simulink model "navigationstates"  (R2013b)
settings: Solver=FixedStepDiscrete  SolverMode=SingleTasking  StartTime=0.0  StopTime=inf  FixedStep=0.002  RelTol=1e-3
libraries: arduinolib x8, simulink x3
settings Model: SimulationMode=external  ExtModeTrigDuration=2  Creator=gcampa  LastModifiedBy=Joshua
settings DataIOCC: SignalLoggingSaveFormat=ModelDataLogs  SaveOutput=off  SaveTime=off
settings OptimizationCC: ExpressionDepthLimit=2147483647  OptimizeModelRefInitCode=on  LifeSpan=1
settings DebuggingCC: SolverPrmCheckMsg=none  MultiTaskDSMMsg=warning  MultiTaskCondExecSysMsg=none  FcnCallInpInsideContextMsg=EnableAllAsWarning  StateNameClashWarn=warning  StrictBusMsg=None
settings HardwareCC: ProdBitPerInt=16  ProdBitPerPointer=16  ProdIntDivRoundTo=Zero  ProdEndianess=LittleEndian  ProdWordSize=8  ProdHWDeviceType=Atmel->AVR
settings RTWCC: SystemTargetFile=realtime.tlc  GenerateMakefile=off  TemplateMakefile=realtime.tmf  Description=Real-Time Toolbox  RTWVerbose=off  ProcessScript=realtime_make_rtw_hook  IncludeERTFirstTime=on
settings CodeAppCC: CustomSymbolStrType=$N$R$M  InternalIdentifier=Classic
settings STFCustomTargetCC: TargetLibSuffix=.a  CodeReplacementLibrary=None  GenerateSampleERTMain=on  ERTCustomFileBanners=on  SupportNonInlinedSFcns=off  SupportVariableSizeSignals=on  MATLABClassNameForMDSCustomization=Simulink.SoftwareTarget.ERTCustomization  GRTInterface=off  SystemTargetFile=realtime.tlc
settings ERTTargetCC: GenerateSampleERTMain=on  ParMdlRefBuildCompliant=off  CompOptLevelCompliant=off  ConcurrentExecutionCompliant=off  CombineOutputUpdateFcns=off  ERTFirstTimeCompliant=off  SupportContinuousTime=on  SupportVariableSizeSignals=on  ModelStepFunctionPrototypeControlCompliant=off  CPPClassGenCompliant=off  ExtModeTransport=3  ExtModeMexFile=ext_serial_win32_comm  ExtModeMexArgs=0 1 9600  InlinedParameterPlacement=NonHierarchical  ERTSrcFileBannerTemplate=realtime_code_template.cgt  ERTHdrFileBannerTemplate=realtime_code_template.cgt  ERTDataSrcFileTemplate=realtime_code_template.cgt  ERTDataHdrFileTemplate=realtime_code_template.cgt  ERTCustomFileTemplate=realtime_file_process.tlc

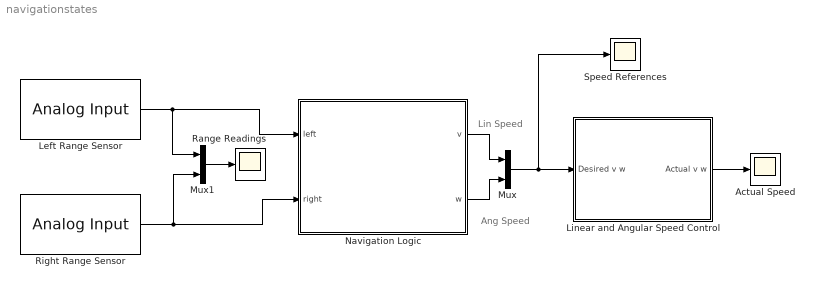
== system navigationstates ==
  note: Ang Speed
  note: Lin Speed
  Actual Speed : Scope
      settings: YMin=34.7  YMax=36
  Left Range Sensor : arduinolib/Analog Input  pinNumber=1  sampleTime=0.05
  Linear and Angular Speed Control : Subsystem
  Mux : Mux  Inputs=2
  Mux1 : Mux  Inputs=2
  Navigation Logic : Stateflow chart  TreatAsAtomicUnit=on
  Range Readings : Scope
      settings: YMin=34.7  YMax=36  SaveName=ScopeData3
  Right Range Sensor : arduinolib/Analog Input  pinNumber=0  sampleTime=0.05
  Speed References : Scope
      settings: YMin=34.7  YMax=36  SaveName=ScopeData2
  wires:
  Navigation Logic/1(v) -> Mux/1
  Mux/1 -> Speed References/1, Linear and Angular Speed Control/1(Desired v w)
  Linear and Angular Speed Control/1(Actual v w) -> Actual Speed/1
  Navigation Logic/2(w) -> Mux/2
  Right Range Sensor/1 -> Navigation Logic/2(right), Mux1/2
  Left Range Sensor/1 -> Navigation Logic/1(left), Mux1/1
  Mux1/1 -> Range Readings/1

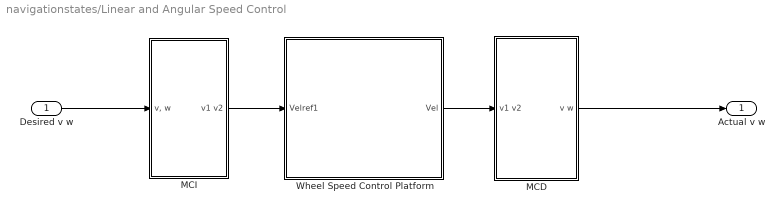
== system navigationstates/Linear and Angular Speed Control ==
  Desired v w : Inport
  MCD : Subsystem
  MCI : Subsystem  mask{d=0.22}
      mask prompts: d "Distancia entre ruedas"
  Wheel Speed Control Platform : Subsystem
      mask Display: image('imagen_robot.png')
  Actual v w : Outport
  wires:
  Wheel Speed Control Platform/1(Vel) -> MCD/1(v1 v2)
  MCD/1(v w) -> Actual v w/1
  MCI/1(v1 v2) -> Wheel Speed Control Platform/1(Velref1)
  Desired v w/1 -> MCI/1("v, w")

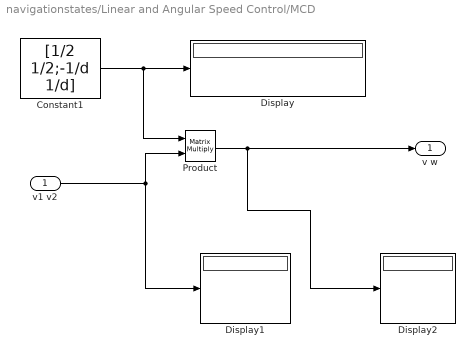
== system navigationstates/Linear and Angular Speed Control/MCD ==
  v1 v2 : Inport
  Constant1 : Constant  Value=[1/2 1/2;-1/d 1/d]  VectorParams1D=off  mask{d=0.22}
      mask prompts: d "distancia"
  Display : Display
  Display1 : Display
  Display2 : Display
  Product : Product  Multiplication=Matrix(*)
  v w : Outport
  wires:
  v1 v2/1 -> Product/2, Display1/1
  Constant1/1 -> Product/1, Display/1
  Product/1 -> v w/1, Display2/1

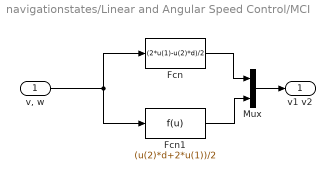
== system navigationstates/Linear and Angular Speed Control/MCI ==
  "v, w" : Inport
  Fcn : Fcn  Expr=(2*u(1)-u(2)*d)/2
  Fcn1 : Fcn  Expr=(u(2)*d+2*u(1))/2
  Mux : Mux  Inputs=2
  v1 v2 : Outport
  wires:
  Fcn/1 -> Mux/1
  Fcn1/1 -> Mux/2
  "v, w"/1 -> Fcn/1, Fcn1/1
  Mux/1 -> v1 v2/1

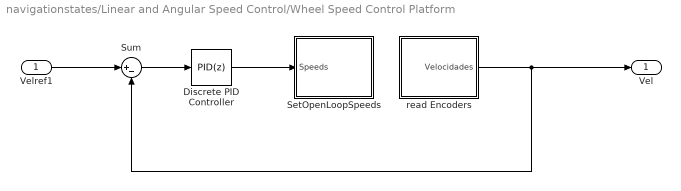
== system navigationstates/Linear and Angular Speed Control/Wheel Speed Control Platform ==
  Velref1 : Inport
  Discrete PID Controller : simulink/Continuous/PID Controller  Controller=PID  TimeDomain=Discrete-time  SampleTime=-1  IntegratorMethod=Forward Euler  FilterMethod=Forward Euler  Form=Parallel  P=1  I=2  D=0  N=100  InitialConditionSource=internal  InitialConditionForIntegrator=0  InitialConditionForFilter=0  ExternalReset=none  LimitOutput=off  UpperSaturationLimit=inf  LowerSaturationLimit=-inf  LinearizeAsGain=off  AntiWindupMode=none  Kb=1  TrackingMode=off  Kt=1  PParamMin=[]  PParamMax=[]  IParamMin=[]  IParamMax=[]  DParamMin=[]  DParamMax=[]  NParamMin=[]  NParamMax=[]  KbParamMin=[]  KbParamMax=[]  KtParamMin=[]  KtParamMax=[]  POutMin=[]  POutMax=[]  IOutMin=[]  IOutMax=[]  DOutMin=[]  DOutMax=[]  NOutMin=[]  NOutMax=[]  KbOutMin=[]  KbOutMax=[]  KtOutMin=[]  KtOutMax=[]  IntegratorOutMin=[]  IntegratorOutMax=[]  FilterOutMin=[]  FilterOutMax=[]  SumOutMin=[]  SumOutMax=[]  SumI1OutMin=[]  SumI1OutMax=[]  SumI2OutMin=[]  SumI2OutMax=[]  SumI3OutMin=[]  SumI3OutMax=[]  SumDOutMin=[]  SumDOutMax=[]  SaturationOutMin=[]  SaturationOutMax=[]  IntegratorContinuousStateAttributes=''  IntegratorStateMustResolveToSignalObject=off  IntegratorRTWStateStorageClass=Auto  FilterContinuousStateAttributes=''  FilterStateMustResolveToSignalObject=off  FilterRTWStateStorageClass=Auto
  SetOpenLoopSpeeds : Subsystem
  Sum : Sum  Inputs=|+-
  read Encoders : Subsystem
  Vel : Outport
  wires:
  Discrete PID Controller/1 -> SetOpenLoopSpeeds/1(Speeds)
  Velref1/1 -> Sum/1
  Sum/1 -> Discrete PID Controller/1
  read Encoders/1(Velocidades) -> Vel/1, Sum/2

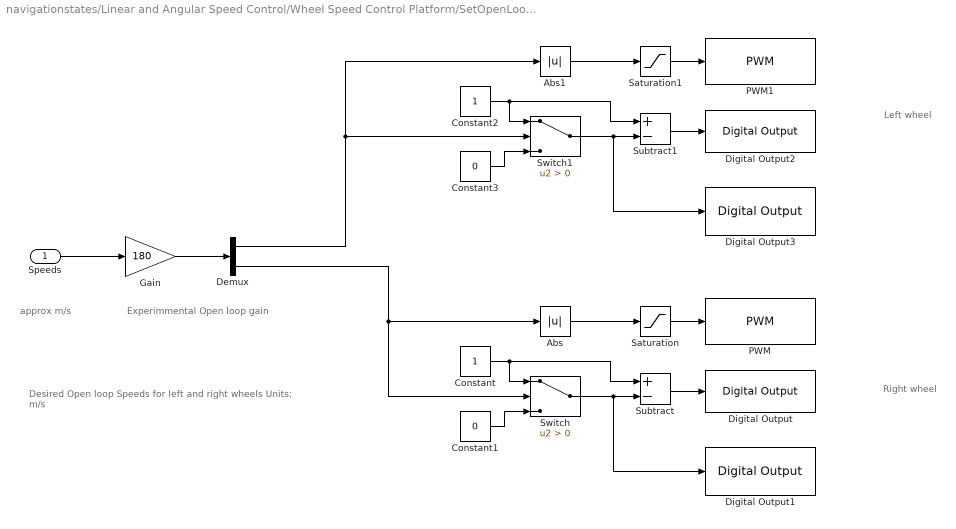
== system navigationstates/Linear and Angular Speed Control/Wheel Speed Control Platform/SetOpenLoopSpeeds ==
  note: Right wheel
  note: Left wheel
  note: approx m/s
  note: Experimmental
      | Open loop gain
  note: Desired Open loop Speeds for left and right wheels
      | Units: m/s
  Speeds : Inport
  Abs : Abs
  Abs1 : Abs
  Constant : Constant
  Constant1 : Constant  Value=0
  Constant2 : Constant
  Constant3 : Constant  Value=0
  Demux : Demux  Outputs=2
  Digital Output : arduinolib/Digital Output  pinNumber=11
  Digital Output1 : arduinolib/Digital Output  pinNumber=12
  Digital Output2 : arduinolib/Digital Output  pinNumber=9
  Digital Output3 : arduinolib/Digital Output  pinNumber=10
  Gain : Gain  Gain=180
  PWM : arduinolib/PWM  pinNumber=13
  PWM1 : arduinolib/PWM  pinNumber=8
  Saturation : Saturate  UpperLimit=255  LowerLimit=0  OutDataTypeStr=uint8
  Saturation1 : Saturate  UpperLimit=255  LowerLimit=0  OutDataTypeStr=uint8
  Subtract : Sum  Inputs=+-
  Subtract1 : Sum  Inputs=+-
  Switch : Switch  Criteria=u2 > Threshold
  Switch1 : Switch  Criteria=u2 > Threshold
  wires:
  Speeds/1 -> Gain/1
  Abs/1 -> Saturation/1
  Gain/1 -> Demux/1
  Constant/1 -> Subtract/1, Switch/1
  Constant1/1 -> Switch/3
  Switch/1 -> Digital Output1/1, Subtract/2
  Subtract/1 -> Digital Output/1
  Saturation/1 -> PWM/1
  Abs1/1 -> Saturation1/1
  Constant2/1 -> Switch1/1, Subtract1/1
  Constant3/1 -> Switch1/3
  Switch1/1 -> Subtract1/2, Digital Output3/1
  Subtract1/1 -> Digital Output2/1
  Saturation1/1 -> PWM1/1
  Demux/1 -> Switch1/2, Abs1/1
  Demux/2 -> Switch/2, Abs/1

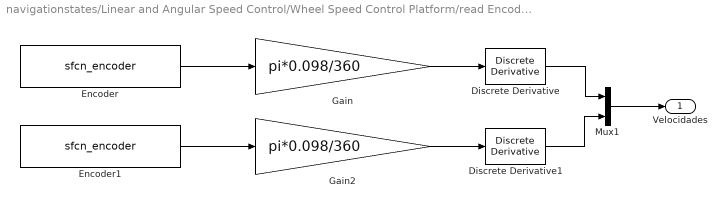
== system navigationstates/Linear and Angular Speed Control/Wheel Speed Control Platform/read Encoders ==
  Discrete Derivative : simulink/Discrete/Discrete Derivative  gainval=1.0  ICPrevScaledInput=0.0  InputProcessing=Inherited  OutMin=[]  OutMax=[]  OutDataType=fixdt(1, 16)  OutScaling=2^-10  DoSatur=off
  Discrete Derivative1 : simulink/Discrete/Discrete Derivative  gainval=1.0  ICPrevScaledInput=0.0  InputProcessing=Inherited  OutMin=[]  OutMax=[]  OutDataType=fixdt(1, 16)  OutScaling=2^-10  DoSatur=off
  Encoder : S-Function  InitFcn=try, set_param(gcb,'FunctionName','sfcn_encoder'), end  FunctionName=sfcn_encoder  Parameters=uint8(0),uint8(3),uint8(2)  SFunctionModules=sfcn_encoder_wrapper  EnableBusSupport=off  mask(S-Function Builder){}
      mask init:
      | val = [[.9  0.75 0.75 1 1 .9 .9 1]',[1 1 0.75 0.75 .9 .9 1 .9]'];try , sys = get_param(gcb,'SfunBuilderFcnName');if isempty(sys), sys = get_param(gcb,'FunctionName'); end,catch, sys = get_param(gcb,'FunctionName'); end
      settings: CopyFcn=set_param(gcbh,'LinkStatus','none')  PreSaveFcn=try, set_param(gcb,'FunctionName','sfcn_encoder'), end  OpenFcn=sfunctionwizard(gcbh)
      mask Display: plot(val(:,1),val(:,2)),disp(sys), port_label('output',1,'pos')
  Encoder1 : S-Function  InitFcn=try, set_param(gcb,'FunctionName','sfcn_encoder'), end  FunctionName=sfcn_encoder  Parameters=uint8(1),uint8(19),uint8(18)  SFunctionModules=sfcn_encoder_wrapper  EnableBusSupport=off  mask(S-Function Builder){}
      mask init: same as navigationstates/Linear and Angular Speed Control/Wheel Speed Control Platform/read Encoders/Encoder
      settings: CopyFcn=set_param(gcbh,'LinkStatus','none')  PreSaveFcn=try, set_param(gcb,'FunctionName','sfcn_encoder'), end  OpenFcn=sfunctionwizard(gcbh)
      mask Display: plot(val(:,1),val(:,2)),disp(sys), port_label('output',1,'pos')
  Gain : Gain  Gain=pi*0.098/360  OutDataTypeStr=double
  Gain2 : Gain  Gain=pi*0.098/360  OutDataTypeStr=double
  Mux1 : Mux  Inputs=2
  Velocidades : Outport
  wires:
  Gain2/1 -> Discrete Derivative1/1
  Gain/1 -> Discrete Derivative/1
  Encoder/1 -> Gain/1
  Encoder1/1 -> Gain2/1
  Discrete Derivative1/1 -> Mux1/2
  Discrete Derivative/1 -> Mux1/1
  Mux1/1 -> Velocidades/1

== stateflow chart navigationstates/Navigation Logic ==
  state Stopped
    en:
    v=0;
    w=0;
  state Forward
    en:
    v=0.5;
    w=0;
  state Avoid
    en:
    v=0;
    w=0.5;
  (default) -> Stopped
  Stopped -> Forward : [(left<400) && (right<400)]
  Avoid -> Stopped [order 1] : after(4,sec)
  Forward -> Avoid : [(left>400) || (right>400)]
  Avoid -> Forward [order 2] : [(left<400) && (right<400)]
  data: v output double; w output double; left input; right input
